simulink model "Neurofeedback_ErrorFunction"  (R2021a)
settings: Solver=VariableStepAuto  StartTime=0.0  StopTime=1  RelTol=1e-3
settings Model: Creator=mariodelossantos  LastModifiedBy=mdls3

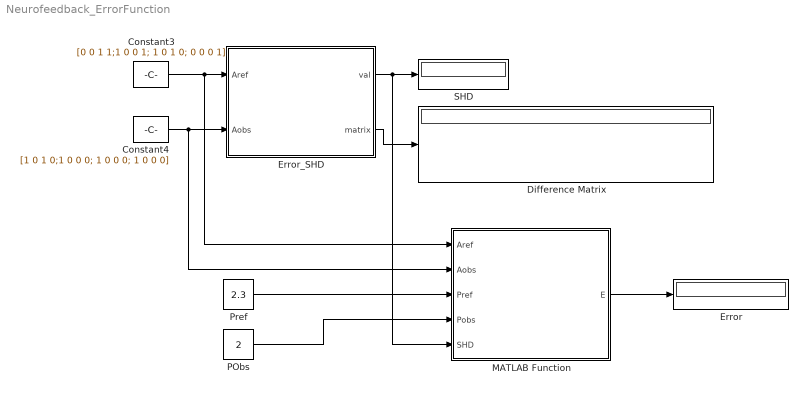
== system Neurofeedback_ErrorFunction ==
  Constant3 : Constant  Value=[0 0 1 1;1 0 0 1; 1 0 1 0; 0 0 0 1]
  Constant4 : Constant  Value=[1 0 1 0;1 0 0 0; 1 0 0 0; 1 0 0 0]
  Difference Matrix : Display
  Error : Display
  Error_SHD : MATLAB Function  TreatAsAtomicUnit=on
  MATLAB Function : MATLAB Function  TreatAsAtomicUnit=on
  PObs : Constant  Value=2
  Pref : Constant  Value=2.3
  SHD : Display
  wires:
  Constant4/1 -> MATLAB Function/2(Aobs), Error_SHD/2(Aobs)
  Error_SHD/1(val) -> MATLAB Function/5(SHD), SHD/1
  Error_SHD/2(matrix) -> Difference Matrix/1
  Constant3/1 -> MATLAB Function/1(Aref), Error_SHD/1(Aref)
  MATLAB Function/1(E) -> Error/1
  Pref/1 -> MATLAB Function/3(Pref)
  PObs/1 -> MATLAB Function/4(Pobs)

== matlab function Neurofeedback_ErrorFunction/Error_SHD ==
  data: Aref input; val output; Aobs input; matrix output
function [val,matrix]=SHD(Aref,Aobs)

val = sum(sum(xor(Aref,Aobs)));
matrix = xor(Aref,Aobs);

== matlab function Neurofeedback_ErrorFunction/MATLAB Function ==
  data: Aref input; E output; Aobs input; Pref input; Pobs input; SHD input
function E  = ErrorFunction(Aref,Aobs,Pref,Pobs,SHD)
    w1 = 0.4; %Use whatever values you like most. Threshold 

    w2 = 1 - w1;

    assert(all(size(Aref) == size(Aobs)));

    assert(size(Aref,1) == size(Aref,2));

    nChannels = size(Aref,1);

    AfullyConnected = ones(nChannels);

    AfullyDisconnected = zeros(nChannels);

    maxDiffSHD = sum(sum(xor(AfullyConnected,AfullyDisconnected))); %SHD

    errA = SHD/maxDiffSHD; %Normalize error in the connectivity

    errP = abs(Pobs-Pref)/abs(Pref);

    
E = w1 * errA + w2 * errP;
